simulink model "MPC_control_ID"  (R2018a)
settings: Solver=FixedStepAuto  StartTime=0  StopTime=Tend  FixedStep=0.001  RelTol=5e-3
model workspace (MAT data in the model file):
  A_mu = 10
  B_reff = 8.386
  Cz = 7766.25
  DCT_Param.Transmission.Ratios = [3.78 2.18 1.43 1.03 0.935 0.84]
  DCT_Param.Transmission.Shaft_Inertia_Odd = 0.0023
  DCT_Param.Transmission.Shaft_Inertia_Even = 0.0009
  DCT_Param.Transmission.Shaft_Inertia_Output = 0.008
  DCT_Param.Transmission.Gear_Inertia = 0.001
  DCT_Param.Transmission.Gear_Efficiency = 0.94
  DCT_Param.Transmission.Gear_Ang_Vel_Thr = 0.01
  DCT_Param.Transmission.Shaft_Velocity_Odd = 0
  DCT_Param.Transmission.Shaft_Velocity_Even = 0
  DCT_Param.Transmission.Shaft_Velocity_Output = 0
  DCT_Param.Transmission.Gear_Initial_Velocity = 0
  DCT_Param.Transmission.Abstract.Compliance = 100000
  DCT_Param.Transmission.Abstract.Damping = 10000
  DCT_Param.Transmission.Abstract.Ratio_Time_Const = 0.05
  DCT_Param.Transmission.Abstract.Shift_Gear_Delay = 25
  DCT_Param.Clutch.Torque_Radius = 130
  DCT_Param.Clutch.Num_Friction_Surfaces = 4
  DCT_Param.Clutch.Engagement_Piston_Area = 0.001
  DCT_Param.Clutch.Kinetic_Friction_Coeff = 0.3
  DCT_Param.Clutch.Static_Friction_Coeff = 0.31
  DCT_Param.Clutch.Derating_Factor = 1
  DCT_Param.Clutch.Clutch_Velocity_Tolerance = 0.001
  DCT_Param.Clutch.Threshold_Pressure = 1
  DCT_Param.Clutch.Drag_Torque_Coeff = 0
  DCT_Param.Dog_Clutch.Max_Torque = 1000
  DCT_Param.Dog_Clutch.Teeth_Mean_Radius = 50
  DCT_Param.Dog_Clutch.Tooth_Height = 10
  DCT_Param.Dog_Clutch.Ring_Hub_Clearance = 3
  DCT_Param.Dog_Clutch.Ring_Stop_Stiffness = 1000000
  DCT_Param.Dog_Clutch.Ring_Stop_Damping = 1000
  DCT_Param.Dog_Clutch.Shift_Linkage_Damping = 100
  DCT_Param.Dog_Clutch.Max_Engage_Velocity = 1000000
  DCT_Param.Dog_Clutch.Tooth_Engage_Overlap = 3
  DCT_Param.Vehicle.Mass = 1600
  DCT_Param.Vehicle.Wheels_Per_Axle = 2
  DCT_Param.Vehicle.Distance_CG_FrontAxle = 1.7
  DCT_Param.Vehicle.Distance_CG_RearAxle = 2
  DCT_Param.Vehicle.Distance_CG_Ground = 0.5
  DCT_Param.Vehicle.Frontal_Area = 3
  DCT_Param.Vehicle.Aero_Drag_Coeff = 0.4
  DCT_Param.Vehicle.Initial_Velocity = 0
  DCT_Param.Vehicle.Final_Drive_Ratio = 3.7
  DCT_Param.Vehicle.Final_Drive_Efficiency = 0.86
  DCT_Param.Vehicle.Final_Drive_Vel_Thresh = 0.01
  DCT_Param.Vehicle.Side_Shaft_Inertia = 0.01
  DCT_Param.Vehicle.Side_Shaft_Initial_Velocity = 0
  DCT_Param.Vehicle.Tire.Radius = 0.312
  DCT_Param.Vehicle.Tire.Inertia = 0.5
  DCT_Param.Vehicle.Tire.Initial_Velocity = 0
  DCT_Param.Vehicle.Tire.Slip_Vel_Thresh = 0.1
  DCT_Param.Vehicle.Tire.Nominal_Vertical_Load = 4000
  DCT_Param.Vehicle.Tire.C_Coeff = 1.685
  DCT_Param.Vehicle.Tire.D_Coeff = [1.21 -0.037]
  DCT_Param.Vehicle.Tire.E_Coeff = [0.344 0.095 -0.02 0]
  DCT_Param.Vehicle.Tire.BCD_Coeff = [21.51 -0.163 0.245]
  DCT_Param.Vehicle.Tire.H_Coeff = [-0.002 0.002]
  DCT_Param.Vehicle.Tire.V_Coeff = [0 0]
  DCT_Param.ICE.Max_Power = 100000
  DCT_Param.ICE.Speed_At_Max_Power = 5500
  DCT_Param.ICE.Max_Speed = 7000
  DCT_Param.ICE.Stall_Speed = 200
  DCT_Param.ICE.Shaft_Inertia = 0.2
  DCT_Param.ICE.Initial_Velocity = 800
  DCT_Param.ICE.Idle_Ref_Spd = 800
  DCT_Param.ICE.Engine_Time_Constant = 0.2
  DCT_Param.ICE.Initial_Normalized_Throttle = 0
  DCT_Param.ICE.Speed_Threshold = 20
  DCT_Param.ICE.FC.Speed_Vector = [0 368.421052632 736.842105263 1105.26315789 1473.68421053 1842.10526316 2210.52631579 2578.94736842 2947.36842105 3315.78947368 3684.21052632 4052.63157895 4421.05263158 4789.47368421 5157.89473684 5526.31578947 5894.73684211 6263.15789474 6631.57894737 7000]
  DCT_Param.ICE.FC.Torque_Vector = [0 10.5263157895 21.0526315789 31.5789473684 42.1052631579 52.6315789474 63.1578947368 73.6842105263 84.2105263158 94.7368421053 105.263157895 115.789473684 126.315789474 136.842105263 147.368421053 157.894736842 168.421052632 178.947368421 189.473684211 200]
  DCT_Param.ICE.FC.Consumption_Table = [0.262945178015 0.225304787522 0.201465019624 0.191425874321 0.195187351614 0.212749451502 0.244112173984 0.289275519063 0.348239486736 0.421004077004 0.507569289868 0.607935125326 ... (400 elements, 20x20)]
  DCT_Param.Shift_Map_Example.Pedal_Positions = [0.1 0.4 0.5 0.9]
  DCT_Param.Shift_Map_Example.Upshift_Speeds = [11  20  26  34.5  43; 14  26  35  44.5  55; 17  31  42  52.5  65; 21  39  52  66.5  80]
  DCT_Param.Shift_Map_Example.Downshift_Speeds = [8.9  17  23.6  32.4  40.8; 11.5  22.7  32  41.6  52.2; 14  27  38.1  50  62; 18  33  48  62.6  76.2]
  DCT_Param.Shift_Map_ORIG.Pedal_Positions = [0.1 0.4 0.5 0.9]
  DCT_Param.Shift_Map_ORIG.Upshift_Speeds = [11.5  23.5  35.5  45.5  55.5; 14.5  26.5  38.5  48.5  58.5; 17.5  29.5  41.5  51.5  61.5; 20.5  32.5  44.5  54.5  64.5]
  DCT_Param.Shift_Map_ORIG.Downshift_Speeds = [8.5  20.5  32.5  42.5  52.5; 11.5  23.5  35.5  45.5  55.5; 14.5  26.5  38.5  48.5  58.5; 17.5  29.5  41.5  51.5  61.5]
  DCT_Param.Shift_Map_OPT.Pedal_Positions = [0.1 0.4 0.5 0.9]
  DCT_Param.Shift_Map_OPT.Upshift_Speeds = [17.8469  29.8469  35.8159  41.2981  46.3004; 19.2469  33.9778  43.9778  53.9778  63.9778; 24.5469  41.9778  62.1778  78.5778  106.9778; 27.5469  59.3778  99.0445  109.0445  119.0445]
  DCT_Param.Shift_Map_OPT.Downshift_Speeds = [14.8469  26.8469  32.8159  38.2981  43.3004; 16.2469  30.9778  40.9778  50.9778  60.9778; 21.5469  38.9778  59.1778  75.5778  103.9778; 24.5469  56.3778  96.0445  106.0445  116.0445]
  DCT_Param.Shift_Map.Pedal_Positions = [0.1 0.4 0.5 0.9]
  DCT_Param.Shift_Map.Upshift_Speeds = [11.5  23.5  35.5  45.5  55.5; 14.5  26.5  38.5  48.5  58.5; 17.5  29.5  41.5  51.5  61.5; 20.5  32.5  44.5  54.5  64.5]
  DCT_Param.Shift_Map.Downshift_Speeds = [8.5  20.5  32.5  42.5  52.5; 11.5  23.5  35.5  45.5  55.5; 14.5  26.5  38.5  48.5  58.5; 17.5  29.5  41.5  51.5  61.5]
  DCT_Param.Control.Clutch.Min_Lock_Pressure = 2000000
  DCT_Param.Control.Clutch.Max_Lock_Pressure = 5000000
  DCT_Param.Control.Clutch.Max_Unlock_Pressure = 500000
  DCT_Param.Control.Engine_Start_RPM = 800
  DCT_Param.Control.Engine_Stop_RPM = 790
  DCT_Param.Control.Mode_Logic_TS = 0.1
  DCT_Param.Control.ICE.Kp = 0.02
  DCT_Param.Control.ICE.Ki = 0.01
  DCT_Param.Control.Gen.Kp = 10
  DCT_Param.Control.Gen.Ki = 3
  DCT_Param.Control.Mot.Kp = 500
  DCT_Param.Control.Mot.Ki = 300
  DCT_Param.Control.Veh_Spd.Kp = 0.02
  DCT_Param.Control.Veh_Spd.Ki = 0.04
  DCT_Param.Driver.Kp = 400
  DCT_Param.Driver.Ki = 0.001
  DCT_Param.Driver.Pedal_Filter_Const = 0.01
  DCT_Param.Dog_Clutches.Pulse_Delay = 50
  DCT_Param.Dog_Clutches.Pulse_Length = 20
  DCT_Param.Animation.Teeth_Ratios = [0.338461538462 0.555555555556 0.916666666667 0.96 1.17948717949 1.92307692308]
  DCT_Param.Animation.Teeth_Ratios_Reverse = [0.458333333333 0.75]
  DCT_Param.Shift_Map_OPT506.Pedal_Positions = [0.1 0.4 0.5 0.9]
  DCT_Param.Shift_Map_OPT506.Upshift_Speeds = [18  30.2  48.3  67.3322  77.3429; 20.1  36.85  66.6178  76.7537  86.7537; 21.1  40.25  71.0189  81.0189  91.7873; 24.1  63.75  80.7523  105.9489  115.9489]
  DCT_Param.Shift_Map_OPT506.Downshift_Speeds = [15  27.2  45.3  64.3322  74.3429; 17.1  33.85  63.6178  73.7537  83.7537; 18.1  37.25  68.0189  78.0189  88.7873; 21.1  60.75  77.7523  102.9489  112.9489]
  DCT_Param.Shift_Map_OPTAbsRea176.Pedal_Positions = [0.1 0.4 0.5 0.9]
  DCT_Param.Shift_Map_OPTAbsRea176.Upshift_Speeds = [17.8469  29.8469  35.7875  44.0901  49.4243; 18.9219  34.1312  45.8256  59.7585  69.7585; 32.1719  43.4585  53.51  103.2151  114.6401; 35.1719  59.2585  99.5217  109.5217  119.5217]
  DCT_Param.Shift_Map_OPTAbsRea176.Downshift_Speeds = [14.8469  26.8469  32.7875  41.0901  46.4243; 15.9219  31.1312  42.8256  56.7585  66.7585; 29.1719  40.4585  50.51  100.2151  111.6401; 32.1719  56.2585  96.5217  106.5217  116.5217]
  D_reff = 0.25826
  Downshift_Speeds = [9.5625  23.0625  36.5625  47.8125  59.0625  68.90625  78.75; 12.9375  26.4375  39.9375  51.1875  62.4375  72.84375  83.25; 16.3125  29.8125  43.3125  54.5625  65.8125  76.78125  87.75; 19.6875  33.1875  46.6875  57.9375  69.1875  80.71875  92.25]
  Pedal_Positions = [0.1 0.4 0.5 0.9]
  SUS.Stiffness = 24000
  SUS.Damping.Constant = 1262
  SUS.Damping.Rebound = [4040 4950 2883 2043]
  SUS.Damping.Compression = [3600 3420 1863 1472]
  SUS.PistonSpeed = [0.05 0.1 0.3 0.6]
  SUS.UnsprungMass.Fr = 21.0693333333
  SUS.UnsprungMass.Rr = 21.0693333333
  Upshift_Speeds = [12.9375  26.4375  39.9375  51.1875  62.4375  72.84375  83.25; 16.3125  29.8125  43.3125  54.5625  65.8125  76.78125  87.75; 19.6875  33.1875  46.6875  57.9375  69.1875  80.71875  92.25; 33  52.5  77.25  100.5  138.75  161.875  185]
  VEH.Mass = 1181
  VEH.StaticNormalFrontLoad.FR = 264.666666667
  VEH.StaticNormalFrontLoad.FL = 264.666666667
  VEH.StaticNormalRearLoad.RR = 322
  VEH.StaticNormalRearLoad.RL = 322
  VEH.WheelBase = 3.075
  VEH.FrontAxlePositionfromCG = 1.515
  VEH.RearAxlePositionfromCG = 1.504
  VEH.HeightCG = 0.134
  VEH.FrontalArea = 2.11
  VEH.DragCoefficient = 0.33
  VEH.NumberOfWheelsPerAxle = 2
  VEH.Thread.FR = 1.705
  VEH.Thread.RR = 1.705
  VEH.PitchMomentInertia = 1922.66666667
  VEH.RollMomentInertia = 432.333333333
  VEH.YawMomentInertia = 2066
  VEH.SteeringRatio = 18
  VEH.TrackWidth = 1.922
  VEH.SprungMass = 1096.72266667
  VEH.InitialLongPosition = 0
  VEH.InitialLatPosition = 3.125
  VEH.InitialVertPosition = 0.0111
  VEH.InitialRollAngle = 0
  VEH.InitialPitchAngle = -0.000732
  VEH.InitialYawAngle = 0
  VEH.InitialLongVel = 0
  VEH.InitialLatVel = 0
  VEH.InitialVertVel = 0
  VEH.InitialRollRate = 0
  VEH.InitialPitchRate = 0
  VEH.InitialYawRate = 0
  V_o = 16.7
  V_xlow = 1
  WH.Tire.Radius.Front = 0.384
  WH.Tire.Radius.Rear = 0.401
  WH.Tire.Sidewall = 0.245
  WH.Tire.RollingResistCoeff = 0.0103
  WH.Tire.Magic.B = 10
  WH.Tire.Magic.C = 1.9
  WH.Tire.Magic.D = 1
  WH.Tire.Magic.E = 0.97
  WH.Tire.Magic.Bx = 12
  WH.Tire.Magic.Cx = 1.9
  WH.Tire.Magic.Dx = 0.72
  WH.Tire.Magic.Ex = 0.95
  WH.Tire.Magic.By = 12
  WH.Tire.Magic.Cy = 1.3
  WH.Tire.Magic.Dy = 0.75
  WH.Tire.Magic.Ey = 0.2
  WH.Tire.Front.Ky = 40000
  WH.Tire.Rear.Ky = 40000
  WH.Tire.Kz = 320000
  WH.Tire.Damping = 100
  WH.Inertia = 1.00333333333
  WH.Mass = 11.4333333333
  WH.DampingCoefficient = 0.01
  WH.VelocityTol = 0.1
  a = 1.4
  alpha_max = 1.5
  alpha_min = -1.5
  b = 1.8
  c_zo = 209651
  epsilon = 0.1
  h = 0.134
  path.ISO3888p2.x = [0 2 12 25.5 36.5 49 61]
  path.ISO3888p2.y = [0 0 0 3.725 3.725 0 0]
  path.ISO3888p2.ylb = [1.225 1.225 1.225 4.725 4.725 1.5 1.5]
  path.ISO3888p2.yrb = [-1.225 -1.225 -1.225 2.225 2.225 -1.5 -1.5]
  path.CUSC.x = [10.668 21.336 36.576 54.864 73.152]
  path.CUSC.y = [0 0 5.1816 0 0]
  path.CUSC.ylb = [1.2192 1.2192 7.0104 1.8288 1.8288]
  path.CUSC.yrb = [-1.2192 -1.2192 3.3528 -1.8288 -1.8288]
  pio = 220000
  q_Fcx = 0
  q_Fz2 = 15.4
  q_Fzy = 0
  q_reo = 0.9974
  q_sx1 = -0.007764
  q_sx10 = 0.2824
  q_sx11 = 5.349
  q_sx12 = 0
  q_sx13 = 0
  q_sx14 = 0
  q_sx2 = 1.1915
  q_sx3 = 0.013948
  q_sx4 = 4.912
  q_sx5 = 1.02
  q_sx6 = 22.83
  q_sx7 = 0.7104
  q_sx8 = -0.023393
  q_sx9 = 0.6581
  q_sy1 = 0.00702
  q_sy2 = 0
  q_sy3 = 0.001515
  q_sy4 = 8.514e-05
  q_sy5 = 0
  q_sy6 = 0
  q_sy7 = 0.9008
  q_sy8 = -0.4089
  q_v1 = 0.0007742
  q_v2 = 0.04667
  r_Bx1 = 12.531
  r_Bx2 = 9.532
  r_Bx3 = 0
  r_By1 = 10.615
  r_By2 = 7.705
  r_By3 = 3.433e-06
  r_By4 = 0
  r_Cx1 = 1.019
  r_Cy1 = 1.0585
  r_Ex1 = -0.4487
  r_Ex2 = -0.4726
  r_Ey1 = 0.3132
  r_Ey2 = 7.63e-06
  r_Hx1 = 0.0002374
  r_Hy1 = 0.011646
  r_Hy2 = 7.63e-06
  r_Vy1 = 0.05654
  r_Vy2 = 7.63e-06
  r_Vy3 = 0
  r_Vy4 = 99.9
  r_Vy5 = 2
  r_Vy6 = 15.814
  r_o = 0.3135
  vehWidth = 2
  w = 1
undefined symbols (not defined in the file): F, Gd, Hd, JE, JF_part, Ld, M, Np, ro, Tf, Ts, U_max, U_min, XYplot
libraries: simulink x5, sim3dlib x2, autolibutils x1, vehdynlibviscommon x1
(part 1 of 2)
settings Model: ModifiedByFormat=The MathWorks, Inc.  Creator=The MathWorks, Inc.  LastModifiedBy=The MathWorks, Inc.
settings SolverCC: ZeroCrossAlgorithm=Adaptive  DecoupledContinuousIntegration=on  MinimalZcImpactIntegration=on
settings DebuggingCC: SignalInfNanChecking=error  ArtificialAlgebraicLoopMsg=none  IgnoredZcDiagnostic=none  ModelReferenceExtraNoncontSigs=none
settings ModelReferenceCC: UpdateModelReferenceTargets=IfOutOfDate  EnableParallelModelReferenceBuilds=on  ModelReferenceMinAlgLoopOccurrences=on  PropagateSignalLabelsOutOfModel=off
settings RTWCC: BuildConfiguration=Faster Runs

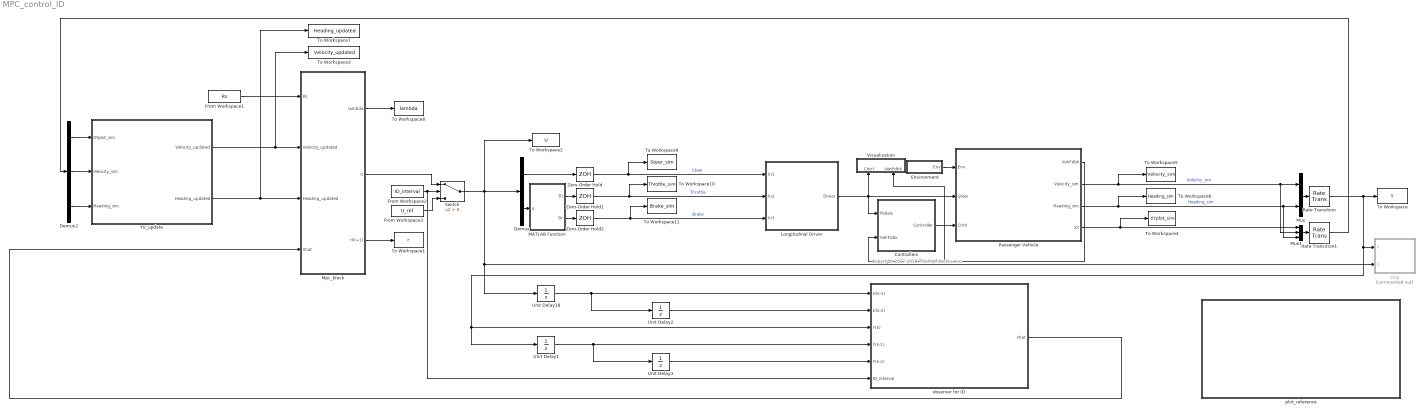
== system MPC_control_ID ==
  note: Copyright 2017-2018 The MathWorks, Inc.
  Controllers : Subsystem
      mask Display: image('SystemControllers.png')
  Demux : Demux  Outputs=2
  Demux2 : Demux  Outputs=3
  Environment : Subsystem  TreatAsAtomicUnit=on
      mask Display: disp('Environment')
  From Workspace1 : FromWorkspace  VariableName=Rs  SampleTime=Ts
  From Workspace2 : FromWorkspace  VariableName=ID_interval  SampleTime=Ts
  From Workspace3 : FromWorkspace  VariableName=U_ref  SampleTime=Ts
  Longitudinal Driver : Subsystem  SystemSampleTime=Tf  VariantControl=0
      mask Display: image('longitudinal_driver_pedals.png');
  MATLAB Function : MATLAB Function  TreatAsAtomicUnit=on  SystemSampleTime=Ts
  Mpc_block : Subsystem  TreatAsAtomicUnit=on  SystemSampleTime=Ts
  Mux : Mux  Inputs=2
  Mux1 : Mux  Inputs=3
  Passenger Vehicle : Subsystem  TreatAsAtomicUnit=on
      settings: MinAlgLoopOccurrences=on
      mask Display: image('PassengerVehicle.png')
  Rate Transition : RateTransition  OutPortSampleTime=Ts
  Rate Transition1 : RateTransition  OutPortSampleTime=Ts
  Switch : Switch  Criteria=u2 > Threshold
  To Workspace : ToWorkspace  VariableName=Y  SampleTime=Ts
  To Workspace1 : ToWorkspace  VariableName=r  SampleTime=Ts
  To Workspace10 : ToWorkspace  VariableName=Throttle_sim  SampleTime=Ts
  To Workspace11 : ToWorkspace  VariableName=Brake_sim  SampleTime=Ts
  To Workspace2 : ToWorkspace  VariableName=U  SampleTime=Ts
  To Workspace3 : ToWorkspace  VariableName=Velocity_updated  SampleTime=Ts
      settings: Save2DSignal=2-D array (concatenate along first dimension)
  To Workspace4 : ToWorkspace  VariableName=XYplot_sim  SampleTime=Ts
  To Workspace5 : ToWorkspace  VariableName=Velocity_sim  SampleTime=Ts
  To Workspace6 : ToWorkspace  VariableName=Heading_sim  SampleTime=Ts
  To Workspace7 : ToWorkspace  VariableName=Heading_updated  SampleTime=Ts
      settings: Save2DSignal=2-D array (concatenate along first dimension)
  To Workspace8 : ToWorkspace  VariableName=lambda  SampleTime=Ts
  To Workspace9 : ToWorkspace  VariableName=Steer_sim  SampleTime=Ts
  Unit Delay1 : UnitDelay  InitialCondition=ro  SampleTime=Ts
  Unit Delay18 : UnitDelay  InitialCondition=[0;0]  SampleTime=Ts
  Unit Delay2 : UnitDelay  InitialCondition=[0;0]  SampleTime=Ts
  Unit Delay3 : UnitDelay  InitialCondition=ro  SampleTime=Ts
  Visualization : Subsystem  TreatAsAtomicUnit=on
      mask Display: disp('Visualization')
  YV_update : Subsystem  TreatAsAtomicUnit=on
  Zero-Order Hold : ZeroOrderHold  SampleTime=Tf
  Zero-Order Hold1 : ZeroOrderHold  SampleTime=Tf
  Zero-Order Hold2 : ZeroOrderHold  SampleTime=Tf
  observer for ID : Subsystem
  plot_reference : Subsystem
      settings: MinAlgLoopOccurrences=on
  stop : Subsystem  Commented=on
  wires:
  Longitudinal Driver/1(Driver) -> Passenger Vehicle/2(Steer), Controllers/1(Pedals), Visualization/1(Cntrl)
  Environment/1(Env) -> Passenger Vehicle/1(Env)
  Controllers/1(Controller) -> Passenger Vehicle/3(Cntrl)
  Passenger Vehicle/1(VehFdbk) -> Controllers/2(VehFdbk), Visualization/2(VehFdbk)
  Demux/1 -> Zero-Order Hold/1
  MATLAB Function/1(Th) -> Zero-Order Hold1/1
  MATLAB Function/2(Br) -> Zero-Order Hold2/1
  Passenger Vehicle/3(Heading_sim) -> To Workspace6/1, Mux/2, Mux1/3  "Heading_sim"
  Mux/1 -> Rate Transition/1
  Demux/2 -> MATLAB Function/1(u)
  Zero-Order Hold/1 -> To Workspace9/1, Longitudinal Driver/1(In1)  "Steer"
  Zero-Order Hold1/1 -> To Workspace10/1, Longitudinal Driver/2(In2)  "Throttle"
  Zero-Order Hold2/1 -> To Workspace11/1, Longitudinal Driver/3(In3)  "Brake"
  Passenger Vehicle/2(Velocity_sim) -> To Workspace5/1, Mux/1, Mux1/2  "Velocity_sim"
  YV_update/2(Heading_updated) -> Mpc_block/3(Heading_updated), To Workspace7/1
  YV_update/1(Velocity_updated) -> Mpc_block/2(Velocity_updated), To Workspace3/1
  Demux2/2 -> YV_update/2(Velocity_sim)
  Mux1/1 -> Rate Transition1/1
  Demux2/1 -> YV_update/1(XYplot_sim)
  Demux2/3 -> YV_update/3(Heading_sim)
  Rate Transition1/1 -> Demux2/1
  From Workspace1/1 -> Mpc_block/1(Rs)
  Passenger Vehicle/4(XY) -> To Workspace4/1, Mux1/1
  observer for ID/1(xhat) -> Mpc_block/4(Xhat)
  Rate Transition/1 -> stop/1(Y), Unit Delay1/1, observer for ID/3(Y(k)), To Workspace/1
  Mpc_block/1(lambda) -> To Workspace8/1
  From Workspace2/1 -> Switch/2, observer for ID/6(ID_interval)
  Mpc_block/2(U) -> Switch/1
  Switch/1 -> To Workspace2/1, Demux/1, stop/2(U), Unit Delay18/1
  Unit Delay18/1 -> Unit Delay2/1, observer for ID/1(U(k-1))
  Unit Delay1/1 -> Unit Delay3/1, observer for ID/4(Y(k-1))
  Mpc_block/3(r(k+1)) -> To Workspace1/1
  Unit Delay2/1 -> observer for ID/2(U(k-2))
  Unit Delay3/1 -> observer for ID/5(Y(k-2))
  From Workspace3/1 -> Switch/3

== system MPC_control_ID/Controllers ==
  Pedals : Inport
  VehFdbk : Inport  Port=2
  Brake Controller : Subsystem
  Bus Creator : BusCreator  Inputs=1
  Bus Creator1 : BusCreator  Inputs=1
  Bus Creator2 : BusCreator  Inputs=1
  Bus Creator3 : BusCreator  Inputs=3
  Bus Selector : BusSelector  OutputSignals=Body.xdot,Wheels.kappa
  Bus Selector1 : BusSelector  OutputSignals=Driveline.EngSpd,Driveline.PropShftSpd
  Bus Selector2 : BusSelector  OutputSignals=Accel,Brake
  ECU : Subsystem
  Transmission Controller : Subsystem
  Controller : Outport
  wires:
  Transmission Controller/1(Gear) -> Bus Creator1/1  "GearCmd"
  Bus Selector/2 -> Brake Controller/3(kappa)  "<kappa>"
  ECU/1(Trq Cmd) -> Bus Creator/1  "EngTrqCmd"
  Brake Controller/1(PCmd) -> Bus Creator2/1  "PrsCmd"
  VehFdbk/1 -> Bus Selector/1, Bus Selector1/1
  Bus Selector/1 -> Brake Controller/2(xdot)  "<xdot>"
  Bus Selector1/1 -> Transmission Controller/2(EngSpd)  "<EngSpd>"
  Bus Selector1/2 -> Transmission Controller/3(PropShaftSpd)  "<PropShftSpd>"
  Pedals/1 -> Bus Selector2/1
  Bus Selector2/1 -> Transmission Controller/1(Acc), ECU/1(<Accel>)  "<Accel>"
  Bus Selector2/2 -> Brake Controller/1(BrkPrsCmd)  "<Brake>"
  Bus Creator/1 -> Bus Creator3/1  "ECU"
  Bus Creator1/1 -> Bus Creator3/2  "Transmission"
  Bus Creator2/1 -> Bus Creator3/3  "Brake"
  Bus Creator3/1 -> Controller/1  "Controller"

== system MPC_control_ID/Environment ==
  Bus Creator : BusCreator  Inputs=4
  Bus Creator1 : BusCreator  Inputs=2
  Bus Creator2 : BusCreator  Inputs=4
  Bus Creator3 : BusCreator  Inputs=2
  Constant1 : Constant  Value=zeros(4,1)
  Constant3 : Constant  Value=0
  Constant4 : Constant  Value=0
  Constant5 : Constant  Value=0
  Demux : Demux
  Demux1 : Demux
  Friction : Constant  Value=ones(4,1).*1
  Vector Concatenate : Concatenate  NumInputs=3
  Env : Outport
  wires:
  Constant1/1 -> Demux/1
  Bus Creator2/1 -> Bus Creator3/2  "mu"
  Bus Creator/1 -> Bus Creator3/1  "z"
  Demux/2 -> Bus Creator/2  "G_FR_z"
  Demux/3 -> Bus Creator/3  "G_RL_z"
  Constant5/1 -> Vector Concatenate/3  "Z"
  Demux/1 -> Bus Creator/1  "G_FL_z"
  Vector Concatenate/1 -> Bus Creator1/1  "Wind"
  Constant3/1 -> Vector Concatenate/1  "X"
  Demux/4 -> Bus Creator/4  "G_RR_z"
  Constant4/1 -> Vector Concatenate/2  "Y"
  Demux1/3 -> Bus Creator2/3  "mu_RL"
  Demux1/4 -> Bus Creator2/4  "mu_RR"
  Demux1/2 -> Bus Creator2/2  "mu_FR"
  Demux1/1 -> Bus Creator2/1  "mu_FL"
  Friction/1 -> Demux1/1
  Bus Creator3/1 -> Bus Creator1/2  "Gnd"
  Bus Creator1/1 -> Env/1

== system MPC_control_ID/Longitudinal Driver ==
  In1 : Inport  SampleTime=Tf
  In2 : Inport  Port=2  SampleTime=Tf
  In3 : Inport  Port=3  SampleTime=Tf
  Bus Creator1 : BusCreator  Inputs=3
  Driver : Outport
  wires:
  Bus Creator1/1 -> Driver/1
  In2/1 -> Bus Creator1/2  "Accel"
  In3/1 -> Bus Creator1/3  "Brake"
  In1/1 -> Bus Creator1/1  "Steer"

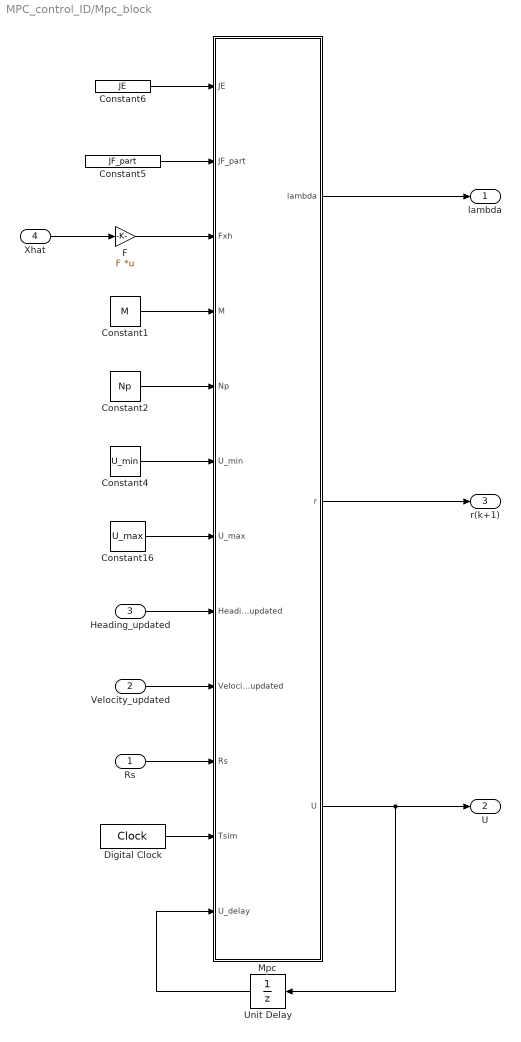
== system MPC_control_ID/Mpc_block ==
  Rs : Inport  SampleTime=Ts  LockScale=on
  Velocity_updated : Inport  Port=2  SampleTime=Ts
  Heading_updated : Inport  Port=3  SampleTime=Ts  LockScale=on
  Xhat : Inport  Port=4
  Constant1 : Constant  Value=M  VectorParams1D=off  SampleTime=-1
  Constant16 : Constant  Value=U_max  VectorParams1D=off  SampleTime=-1
  Constant2 : Constant  Value=Np  SampleTime=-1
  Constant4 : Constant  Value=U_min  VectorParams1D=off  SampleTime=-1
  Constant5 : Constant  Value=JF_part  VectorParams1D=off  SampleTime=-1
  Constant6 : Constant  Value=JE  VectorParams1D=off  SampleTime=-1
  Digital Clock : DigitalClock  SampleTime=Ts
  F : Gain  Gain=F  Multiplication=Matrix(K*u) (u vector)
  Mpc : MATLAB Function  TreatAsAtomicUnit=on  SystemSampleTime=Ts
  Unit Delay : UnitDelay  InitialCondition=[0;0]  SampleTime=Ts
  lambda : Outport
  U : Outport  Port=2
  r(k+1) : Outport  Port=3
  wires:
  Unit Delay/1 -> Mpc/12(U_delay)
  Heading_updated/1 -> Mpc/8(Heading_updated)
  Constant1/1 -> Mpc/4(M)
  Mpc/3(U) -> U/1, Unit Delay/1
  Constant2/1 -> Mpc/5(Np)
  Xhat/1 -> F/1
  Rs/1 -> Mpc/10(Rs)
  Constant4/1 -> Mpc/6(U_min)
  Velocity_updated/1 -> Mpc/9(Velocity_updated)
  Constant6/1 -> Mpc/1(JE)
  Mpc/2(r) -> r(k+1)/1
  Digital Clock/1 -> Mpc/11(Tsim)
  Constant16/1 -> Mpc/7(U_max)
  Mpc/1(lambda) -> lambda/1
  F/1 -> Mpc/3(Fxh)
  Constant5/1 -> Mpc/2(JF_part)

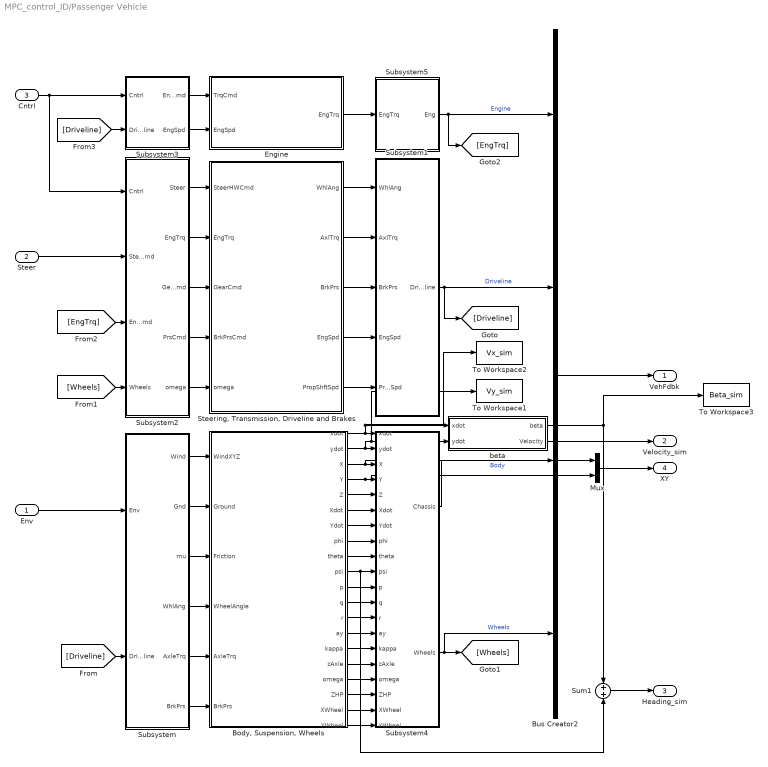
== system MPC_control_ID/Passenger Vehicle ==
  Env : Inport
  Steer : Inport  Port=2
  Cntrl : Inport  Port=3
  "Body, Suspension, Wheels" : Subsystem  Variant=on  OverrideUsingVariant=1
  Bus Creator2 : BusCreator  Inputs=4
  Engine : Subsystem  Variant=on  OverrideUsingVariant=0
  Mux : Mux  Inputs=2
  "Steering, Transmission, Driveline and Brakes" : Subsystem  Variant=on  OverrideUsingVariant=0
  Subsystem : Subsystem
  Subsystem1 : Subsystem
  Subsystem2 : Subsystem
  Subsystem3 : Subsystem
  Subsystem4 : Subsystem
  Subsystem5 : Subsystem
  Sum1 : Sum
  To Workspace1 : ToWorkspace  VariableName=Vy_sim  SampleTime=Ts
  To Workspace2 : ToWorkspace  VariableName=Vx_sim  SampleTime=Ts
  To Workspace3 : ToWorkspace  VariableName=Beta_sim  SampleTime=Ts
  beta : MATLAB Function  TreatAsAtomicUnit=on  SystemSampleTime=Tf
      settings: MinAlgLoopOccurrences=on
  VehFdbk : Outport
  Velocity_sim : Outport  Port=2
  Heading_sim : Outport  Port=3
  XY : Outport  Port=4
  wires:
  Bus Creator2/1 -> VehFdbk/1
  Env/1 -> Subsystem/1(Env)
  Subsystem1/1(Driveline) -> [Driveline], Bus Creator2/2  "Driveline"
  "Steering, Transmission, Driveline and Brakes"/1(WhlAng) -> Subsystem1/1(WhlAng)
  "Steering, Transmission, Driveline and Brakes"/2(AxlTrq) -> Subsystem1/2(AxlTrq)
  "Steering, Transmission, Driveline and Brakes"/3(BrkPrs) -> Subsystem1/3(BrkPrs)
  "Steering, Transmission, Driveline and Brakes"/4(EngSpd) -> Subsystem1/4(EngSpd)
  "Steering, Transmission, Driveline and Brakes"/5(PropShftSpd) -> Subsystem1/5(PropShftSpd)
  Steer/1 -> Subsystem2/2(SteerCmd)
  Cntrl/1 -> Subsystem3/1(Cntrl), Subsystem2/1(Cntrl)
  Subsystem2/1(Steer) -> "Steering, Transmission, Driveline and Brakes"/1(SteerHWCmd)
  Subsystem2/3(GearCmd) -> "Steering, Transmission, Driveline and Brakes"/3(GearCmd)
  Subsystem2/4(PrsCmd) -> "Steering, Transmission, Driveline and Brakes"/4(BrkPrsCmd)
  Subsystem2/5(omega) -> "Steering, Transmission, Driveline and Brakes"/5(omega)
  Engine/1(EngTrq) -> Subsystem5/1("EngTrq ")
  Subsystem2/2(EngTrq) -> "Steering, Transmission, Driveline and Brakes"/2(EngTrq)
  Subsystem3/1(EngTrqCmd) -> Engine/1(TrqCmd)
  Subsystem3/2(EngSpd) -> Engine/2(EngSpd)
  Subsystem4/1(Chassis) -> Bus Creator2/3  "Body"
  Subsystem4/2(Wheels) -> Bus Creator2/4, [Wheels]  "Wheels"
  Subsystem5/1(Eng) -> [EngTrq], Bus Creator2/1  "Engine"
  [Driveline] -> Subsystem/2(Driveline)
  [Wheels] -> Subsystem2/4(Wheels)
  [EngTrq] -> Subsystem2/3(EngTrqCmd)
  [Driveline] -> Subsystem3/2(Driveline)
  "Body, Suspension, Wheels"/19(XWheel) -> Subsystem4/19(XWheel)
  "Body, Suspension, Wheels"/11(p) -> Subsystem4/11(p)
  "Body, Suspension, Wheels"/12(q) -> Subsystem4/12(q)
  "Body, Suspension, Wheels"/7(Ydot) -> Subsystem4/7(Ydot)
  "Body, Suspension, Wheels"/13(r) -> Subsystem4/13(r)
  "Body, Suspension, Wheels"/16(zAxle) -> Subsystem4/16(zAxle)
  "Body, Suspension, Wheels"/8(phi) -> Subsystem4/8(phi)
  "Body, Suspension, Wheels"/3(X) -> Mux/1, Subsystem4/3(X)
  Subsystem/6(BrkPrs) -> "Body, Suspension, Wheels"/6(BrkPrs)
  "Body, Suspension, Wheels"/9(theta) -> Subsystem4/9(theta)
  "Body, Suspension, Wheels"/5(Z) -> Subsystem4/5(Z)
  Subsystem/3(mu) -> "Body, Suspension, Wheels"/3(Friction)
  "Body, Suspension, Wheels"/17(omega) -> Subsystem4/17(omega)
  Subsystem/4(WhlAng) -> "Body, Suspension, Wheels"/4(WheelAngle)
  "Body, Suspension, Wheels"/14(ay) -> Subsystem4/14(ay)
  Subsystem/1(Wind) -> "Body, Suspension, Wheels"/1(WindXYZ)
  Subsystem/2(Gnd) -> "Body, Suspension, Wheels"/2(Ground)
  "Body, Suspension, Wheels"/10(psi) -> Subsystem4/10(psi), Sum1/2
  "Body, Suspension, Wheels"/4(Y) -> Mux/2, Subsystem4/4(Y)
  Subsystem/5(AxleTrq) -> "Body, Suspension, Wheels"/5(AxleTrq)
  "Body, Suspension, Wheels"/18(ZHP) -> Subsystem4/18(ZHP)
  "Body, Suspension, Wheels"/20(YWheel) -> Subsystem4/20(YWheel)
  "Body, Suspension, Wheels"/6(Xdot) -> Subsystem4/6(Xdot)
  "Body, Suspension, Wheels"/15(kappa) -> Subsystem4/15(kappa)
  Mux/1 -> XY/1
  Sum1/1 -> Heading_sim/1
  beta/1(beta) -> To Workspace3/1, Sum1/1
  "Body, Suspension, Wheels"/2(ydot) -> To Workspace1/1, beta/2(ydot), Subsystem4/2(ydot)
  "Body, Suspension, Wheels"/1(xdot) -> To Workspace2/1, beta/1(xdot), Subsystem4/1(xdot)
  beta/2(Velocity) -> Velocity_sim/1

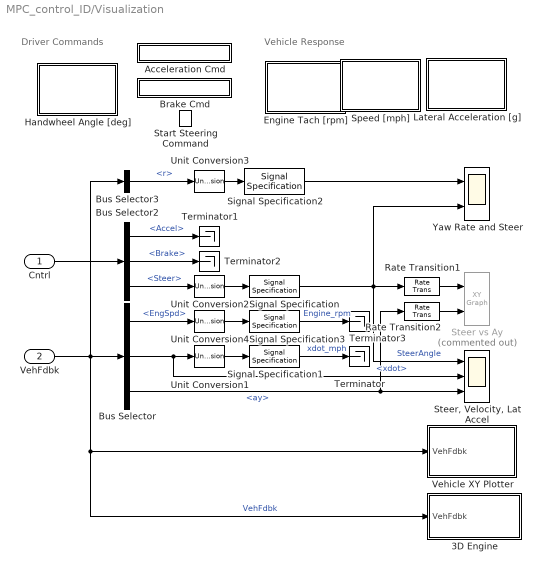
== system MPC_control_ID/Visualization ==
  note: Driver Commands
  note: Vehicle Response
  Cntrl : Inport
  VehFdbk : Inport  Port=2
  3D Engine : Subsystem  Variant=on  OverrideUsingVariant=0  mask(3D Engine){engine3D=Disabled, SceneDesc=Straight road, dt3D=.03}
      mask prompts: engine3D "3D Engine"; SceneDesc "Scene Description:"; dt3D "Engine frame rate, dt3D [s]:"
      mask help: This subsystem contains the interface blocks which permit the display of the vehicle in 3D virtual environment. Enable it to view the simulation progress, disable it to inhibit the display.
      mask init:
      | switch get_param(gcb,'engine3D')
      |     case 'Disabled'
      |         set_param(gcb,'OverrideUsingVariant','0')
      |     case 'Enabled'
      |        set_param(gcb,'OverrideUsingVariant','1')
      |     otherwise
      |        set_param(gcb,'OverrideUsingVariant','0')
      | end
      settings: AttributesFormatString=%<engine3D>
      mask Help: eval('vdynblkshelp(''vdynblksscenecameraray'')');
      mask TypeOptions engine3D: Enabled | Disabled
      mask Callback engine3D:
      | switch get_param(gcb,'engine3D')
      |     case 'Disabled'
      |         set_param(gcb,'OverrideUsingVariant','0')
      |     case 'Enabled'
      |        set_param(gcb,'OverrideUsingVariant','1')
      |     otherwise
      |        set_param(gcb,'OverrideUsingVariant','0')
      | end
      mask TypeOptions SceneDesc:
      | 3D Engine/Simulation 3D Engine
      | 1/SceneDesc
      mask Display: disp('3D Engine')
  Acceleration Cmd : Subsystem  DialogController=hmiCreateDDGDialog  IsWebBlock=on  mask(MWDashboardBlock){webBlockId=2ec56b20-76c2-4aac-ab3d-2dd24ca42fe8, webBlockType=lineargauge, ShowInLibBrowser=on, ShowInitialText=on, HMISrcModelName=[]}
      mask prompts: webBlockId "WebBlock Id"; webBlockType "WebBlock Type"; HMISrcModelName "Source Model"
      mask help: SimulinkHMI:dialogs:LinearGaugeDialogDesc
      mask Help: helpview([docroot '/mapfiles/simulink.map'], 'hmi_linear_gauge')
      mask Display:
      | if strcmp(get_param(bdroot(gcb),'BlockDiagramType'), 'library')
      |     image([(matlabroot) '/toolbox/simulink/hmi/icons/LinearGauge.png']);
      | end
  Brake Cmd : Subsystem  DialogController=hmiCreateDDGDialog  IsWebBlock=on  mask(MWDashboardBlock){webBlockId=d9917a9d-f04e-4f5f-9d8a-619b2f9adbbc, webBlockType=lineargauge, ShowInLibBrowser=on, ShowInitialText=on, HMISrcModelName=[]}
      mask prompts: webBlockId "WebBlock Id"; webBlockType "WebBlock Type"; HMISrcModelName "Source Model"
      mask help: SimulinkHMI:dialogs:LinearGaugeDialogDesc
      mask Help: helpview([docroot '/mapfiles/simulink.map'], 'hmi_linear_gauge')
      mask Display:
      | if strcmp(get_param(bdroot(gcb),'BlockDiagramType'), 'library')
      |     image([(matlabroot) '/toolbox/simulink/hmi/icons/LinearGauge.png']);
      | end
  Bus Selector : BusSelector  OutputSignals=Driveline.EngSpd,Body.xdot,Body.ay
  Bus Selector2 : BusSelector  OutputSignals=Accel,Brake,Steer
  Bus Selector3 : BusSelector  OutputSignals=Body.r
  Engine Tach [rpm] : Subsystem  DialogController=hmiCreateDDGDialog  IsWebBlock=on  mask(MWDashboardBlock){webBlockId=b43bb858-1bc3-4216-8222-68d06605e534, webBlockType=circulargauge, ShowInLibBrowser=on, ShowInitialText=on, HMISrcModelName=[]}
      mask prompts: webBlockId "WebBlock Id"; webBlockType "WebBlock Type"; HMISrcModelName "Source Model"
      mask help: SimulinkHMI:dialogs:CircularGaugeDialogDesc
      mask Help: helpview([docroot '/mapfiles/simulink.map'], 'hmi_gauge')
      mask Display:
      | if strcmp(get_param(bdroot(gcb),'BlockDiagramType'), 'library')
      |     image([(matlabroot) '/toolbox/simulink/hmi/icons/CircularGauge.png']);
      | end
  Handwheel Angle [deg] : Subsystem  DialogController=hmiCreateDDGDialog  IsWebBlock=on  mask(MWDashboardBlock){webBlockId=4efaf655-7637-4550-9856-9a687d94287b, webBlockType=semicirculargauge, ShowInLibBrowser=on, ShowInitialText=on, HMISrcModelName=[]}
      mask prompts: webBlockId "WebBlock Id"; webBlockType "WebBlock Type"; HMISrcModelName "Source Model"
      mask help: SimulinkHMI:dialogs:SemicircularGaugeDialogDesc
      mask Help: helpview([docroot '/mapfiles/simulink.map'], 'hmi_half_gauge')
      mask Display:
      | if strcmp(get_param(bdroot(gcb),'BlockDiagramType'), 'library')
      |     image([(matlabroot) '/toolbox/simulink/hmi/icons/SemicircularGauge.png']);
      | end
  Lateral Acceleration [g] : Subsystem  DialogController=hmiCreateDDGDialog  IsWebBlock=on  mask(MWDashboardBlock){webBlockId=4c84f06f-3c50-4c9f-a814-1d904b0076de, webBlockType=semicirculargauge, ShowInLibBrowser=on, ShowInitialText=on, HMISrcModelName=[]}
      mask prompts: webBlockId "WebBlock Id"; webBlockType "WebBlock Type"; HMISrcModelName "Source Model"
      mask help: SimulinkHMI:dialogs:SemicircularGaugeDialogDesc
      mask Help: helpview([docroot '/mapfiles/simulink.map'], 'hmi_half_gauge')
      mask Display:
      | if strcmp(get_param(bdroot(gcb),'BlockDiagramType'), 'library')
      |     image([(matlabroot) '/toolbox/simulink/hmi/icons/SemicircularGauge.png']);
      | end
  Rate Transition1 : RateTransition
  Rate Transition2 : RateTransition
  Signal Specification : SignalSpecification  Unit=deg
  Signal Specification1 : SignalSpecification  Unit=mph
  Signal Specification2 : SignalSpecification  Unit=deg/s
  Signal Specification3 : SignalSpecification  Unit=rpm
  Speed [mph] : Subsystem  DialogController=hmiCreateDDGDialog  IsWebBlock=on  mask(MWDashboardBlock){webBlockId=6d425e54-616c-4430-b762-4652b407af79, webBlockType=circulargauge, ShowInLibBrowser=on, ShowInitialText=on, HMISrcModelName=[]}
      mask prompts: webBlockId "WebBlock Id"; webBlockType "WebBlock Type"; HMISrcModelName "Source Model"
      mask help: SimulinkHMI:dialogs:CircularGaugeDialogDesc
      mask Help: helpview([docroot '/mapfiles/simulink.map'], 'hmi_gauge')
      mask Display:
      | if strcmp(get_param(bdroot(gcb),'BlockDiagramType'), 'library')
      |     image([(matlabroot) '/toolbox/simulink/hmi/icons/CircularGauge.png']);
      | end
  Start Steering Command : LampBlock  WebBlockId=3552  LabelPosition=Hide
  Steer vs Ay : simulink/Sinks/XY Graph  Commented=on  xmin=-300  xmax=300  ymin=-1.5  ymax=1.5  st=.1
  "Steer, Velocity, Lat Accel" : Scope  NumInputPorts=3
  Terminator{,1..3} (4 alike) : Terminator
  Unit Conversion{1..4} (4 alike) : UnitConversion
  Vehicle XY Plotter : Subsystem  mask(Vehicle XY Plotter){a=VEH.FrontAxlePositionfromCG, b=VEH.RearAxlePositionfromCG, w=VEH.TrackWidth, bufferSize=1024, pltDT=0.1}
      mask prompts: a "Distance to front axle from CG, a [m]:"; b "Distance to rear axle from CG, b [m]:"; w "Track width, w [m]:"; bufferSize "Path buffer sampe size, bufferSize []:"; pltDT "Plot update rate, pltDT [s]:"
      mask help: This block will display a MATLAB figure which indicates the vehicle path, current position and heading velocity.
      mask TypeOptions a: Vehicle XY Plotter/a
      mask TypeOptions b: Vehicle XY Plotter/b
      mask TypeOptions w: Vehicle XY Plotter/w
      mask TypeOptions bufferSize: Vehicle XY Plotter/bufferSize
  Yaw Rate and Steer : Scope  NumInputPorts=2
  wires:
  Unit Conversion3/1 -> Signal Specification2/1
  Bus Selector3/1 -> Unit Conversion3/1  "<r>"
  Signal Specification2/1 -> Yaw Rate and Steer/1
  Unit Conversion4/1 -> Signal Specification3/1
  Signal Specification3/1 -> Terminator3/1  "Engine_rpm"
  Signal Specification/1 -> Yaw Rate and Steer/2, Rate Transition1/1, "Steer, Velocity, Lat Accel"/1  "SteerAngle"
  Bus Selector2/3 -> Unit Conversion2/1  "<Steer>"
  Signal Specification1/1 -> Terminator/1  "xdot_mph"
  Unit Conversion1/1 -> Signal Specification1/1
  Bus Selector/3 -> Rate Transition2/1, "Steer, Velocity, Lat Accel"/3  "<ay>"
  Bus Selector2/1 -> Terminator1/1  "<Accel>"
  Rate Transition1/1 -> Steer vs Ay/1
  Unit Conversion2/1 -> Signal Specification/1
  Bus Selector/2 -> "Steer, Velocity, Lat Accel"/2, Unit Conversion1/1  "<xdot>"
  VehFdbk/1 -> Bus Selector3/1, Bus Selector/1, Vehicle XY Plotter/1(VehFdbk), 3D Engine/1(VehFdbk)  "VehFdbk"
  Cntrl/1 -> Bus Selector2/1
  Rate Transition2/1 -> Steer vs Ay/2
  Bus Selector/1 -> Unit Conversion4/1  "<EngSpd>"
  Bus Selector2/2 -> Terminator2/1  "<Brake>"

== system MPC_control_ID/YV_update ==
  XYplot_sim : Inport
  Velocity_sim : Inport  Port=2
  Heading_sim : Inport  Port=3
  Constant2 : Constant  Value=Ts  SampleTime=Ts
  From Workspace1 : FromWorkspace  VariableName=Tsim  SampleTime=Ts
  From Workspace3 : FromWorkspace  VariableName=XYplot_ref  SampleTime=Ts
  MATLAB Function2 : MATLAB Function  TreatAsAtomicUnit=on  SystemSampleTime=Ts
  Velocity_updated : Outport
  Heading_updated : Outport  Port=2
  wires:
  MATLAB Function2/1(Velocity_updated) -> Velocity_updated/1
  From Workspace3/1 -> MATLAB Function2/1(XYplot_ref)
  MATLAB Function2/2(Heading_updated) -> Heading_updated/1
  From Workspace1/1 -> MATLAB Function2/6(Tsim)
  XYplot_sim/1 -> MATLAB Function2/2(XYplot_sim)
  Velocity_sim/1 -> MATLAB Function2/3(Velocity_sim)
  Heading_sim/1 -> MATLAB Function2/4(Heading_sim)
  Constant2/1 -> MATLAB Function2/5(Ts)

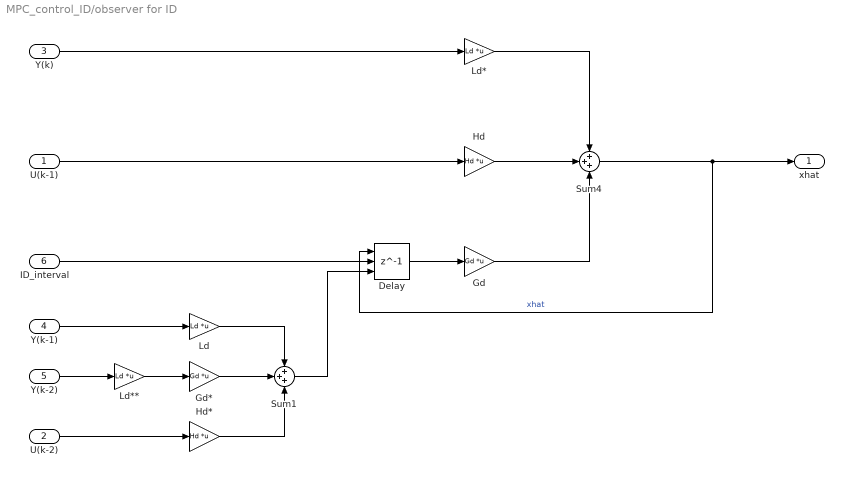
== system MPC_control_ID/observer for ID ==
  U(k-1) : Inport
  U(k-2) : Inport  Port=2
  Y(k) : Inport  Port=3
  Y(k-1) : Inport  Port=4
  Y(k-2) : Inport  Port=5
  ID_interval : Inport  Port=6
  Delay : Delay  DelayLength=1  InitialConditionSource=Input port  InitialCondition=0  ExternalReset=Rising  SampleTime=Ts
      settings: InputPortMap=u0,r5,p4
  Gd : Gain  Gain=Gd  Multiplication=Matrix(K*u) (u vector)
  Gd* : Gain  Gain=Gd  Multiplication=Matrix(K*u) (u vector)
  Hd : Gain  Gain=Hd  Multiplication=Matrix(K*u) (u vector)
  Hd* : Gain  Gain=Hd  Multiplication=Matrix(K*u) (u vector)
  Ld : Gain  Gain=Ld  Multiplication=Matrix(K*u) (u vector)
  Ld* : Gain  Gain=Ld  Multiplication=Matrix(K*u) (u vector)
  Ld** : Gain  Gain=Ld  Multiplication=Matrix(K*u) (u vector)
  Sum1 : Sum  Inputs=+++
  Sum4 : Sum  Inputs=+++
  xhat : Outport
  wires:
  Hd/1 -> Sum4/2
  Ld*/1 -> Sum4/1
  Gd/1 -> Sum4/3
  Sum4/1 -> Delay/1, xhat/1  "xhat"
  Delay/1 -> Gd/1
  Y(k-1)/1 -> Ld/1
  Y(k)/1 -> Ld*/1
  U(k-1)/1 -> Hd/1
  ID_interval/1 -> Delay/2
  Y(k-2)/1 -> Ld**/1
  Ld**/1 -> Gd*/1
  U(k-2)/1 -> Hd*/1
  Ld/1 -> Sum1/1
  Sum1/1 -> Delay/3
  Gd*/1 -> Sum1/2
  Hd*/1 -> Sum1/3

== system MPC_control_ID/plot_reference ==
  Clock : Clock
  Constant : Constant  Value=XYplot  SampleTime=Ts
  MATLAB Function1 : MATLAB Function  TreatAsAtomicUnit=on
  wires:
  Clock/1 -> MATLAB Function1/2(Tsim)
  Constant/1 -> MATLAB Function1/1(XYplot)

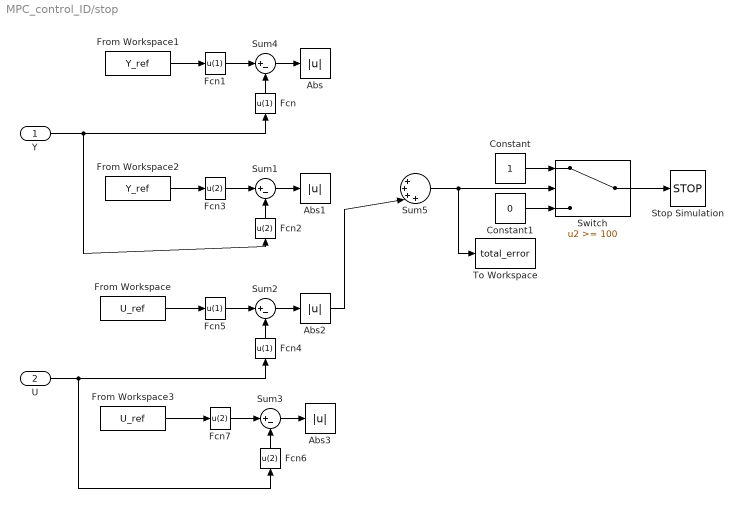
== system MPC_control_ID/stop ==
  Y : Inport
  U : Inport  Port=2
  Abs{,1..3} (4 alike) : Abs
  Constant : Constant
  Constant1 : Constant  Value=0
  Fcn{,1,4..5} (4 alike) : Fcn  Expr=u(1)
  Fcn{2..3,6..7} (4 alike) : Fcn  Expr=u(2)
  From Workspace : FromWorkspace  VariableName=U_ref  SampleTime=Ts
  From Workspace1 : FromWorkspace  VariableName=Y_ref  SampleTime=Ts
  From Workspace2 : FromWorkspace  VariableName=Y_ref  SampleTime=Ts
  From Workspace3 : FromWorkspace  VariableName=U_ref  SampleTime=Ts
  Stop Simulation : Stop
  Sum{1..4} (4 alike) : Sum  Inputs=|+-
  Sum5 : Sum  Inputs=|++++
  Switch : Switch  Threshold=100
  To Workspace : ToWorkspace  VariableName=total_error  SampleTime=Ts
  wires:
  From Workspace1/1 -> Fcn1/1
  Fcn/1 -> Sum4/2
  Fcn1/1 -> Sum4/1
  Sum4/1 -> Abs/1
  Fcn3/1 -> Sum1/1
  Sum1/1 -> Abs1/1
  Y/1 -> Fcn/1, Fcn2/1
  Fcn2/1 -> Sum1/2
  From Workspace2/1 -> Fcn3/1
  Fcn4/1 -> Sum2/2
  Sum2/1 -> Abs2/1
  Fcn5/1 -> Sum2/1
  From Workspace/1 -> Fcn5/1
  U/1 -> Fcn4/1, Fcn6/1
  Sum3/1 -> Abs3/1
  Fcn7/1 -> Sum3/1
  Fcn6/1 -> Sum3/2
  From Workspace3/1 -> Fcn7/1
  Constant/1 -> Switch/1
  Constant1/1 -> Switch/3
  Switch/1 -> Stop Simulation/1
  Sum5/1 -> Switch/2, To Workspace/1
  Abs2/1 -> Sum5/3

== system MPC_control_ID/Controllers/Brake Controller ==
  BrkPrsCmd : Inport
  xdot : Inport  Port=2
  kappa : Inport  Port=3
  Abs : Abs  ZeroCross=off
  Brake Pressure Control : Subsystem  Variant=on  OverrideUsingVariant=0
  Constant1 : Constant  Value=-20
  Gain3 : Gain
  Integrator2 : Integrator  LimitOutput=on  UpperSaturationLimit=1  LowerSaturationLimit=0
  Saturation : Saturate  UpperLimit=1  LowerLimit=0  ZeroCross=off
  Switch1 : Switch  Criteria=u2 > Threshold  Threshold=.1
  Vector Concatenate2 : Concatenate  NumInputs=4
  PCmd : Outport
  wires:
  Constant1/1 -> Switch1/3
  Gain3/1 -> Switch1/1
  Saturation/1 -> Brake Pressure Control/3(<Kappa>)  "Kappa"
  Brake Pressure Control/1(PCmd) -> PCmd/1
  kappa/1 -> Abs/1
  Integrator2/1 -> Vector Concatenate2/4, Vector Concatenate2/3, Vector Concatenate2/2, Vector Concatenate2/1
  xdot/1 -> Brake Pressure Control/2(xdot)
  Abs/1 -> Saturation/1
  Vector Concatenate2/1 -> Brake Pressure Control/1(Pref)  "Reference P"
  BrkPrsCmd/1 -> Switch1/2, Gain3/1
  Switch1/1 -> Integrator2/1

== system MPC_control_ID/Controllers/ECU ==
  <Accel> : Inport
  Acc to Torque Request : Gain  Gain=150
  MATLAB Function : MATLAB Function  TreatAsAtomicUnit=on
  Stop Simulation : Stop
  Trq Cmd : Outport
  wires:
  Acc to Torque Request/1 -> Trq Cmd/1
  <Accel>/1 -> MATLAB Function/1("input ")
  MATLAB Function/2(output) -> Stop Simulation/1
  MATLAB Function/1(input) -> Acc to Torque Request/1

== system MPC_control_ID/Controllers/Transmission Controller ==
  Acc : Inport
  EngSpd : Inport  Port=2  Unit=rad/s
  PropShaftSpd : Inport  Port=3
  10ms Function-Call Generator : simulink/Ports & Subsystems/Function-Call Generator  sample_time=Fcncal_transctrl_Ts  numberOfIterations=1
  Rate Transition{,1..3} (4 alike) : RateTransition
  Signal Specification : SignalSpecification  Unit=rpm
  TCM : Subsystem
  Unit Conversion : UnitConversion
  Gear : Outport
  wires:
  TCM/1(Gear Select) -> Rate Transition3/1
  Rate Transition/1 -> TCM/1(AccCmd)
  10ms Function-Call Generator/1 -> TCM/Trigger
  Acc/1 -> Rate Transition/1
  PropShaftSpd/1 -> Rate Transition2/1
  Rate Transition1/1 -> TCM/2(EngSpd)
  Rate Transition2/1 -> TCM/3(VehSpdFdbk)
  Rate Transition3/1 -> Gear/1
  Unit Conversion/1 -> Signal Specification/1
  Signal Specification/1 -> Rate Transition1/1  "EngSpd"
  EngSpd/1 -> Unit Conversion/1

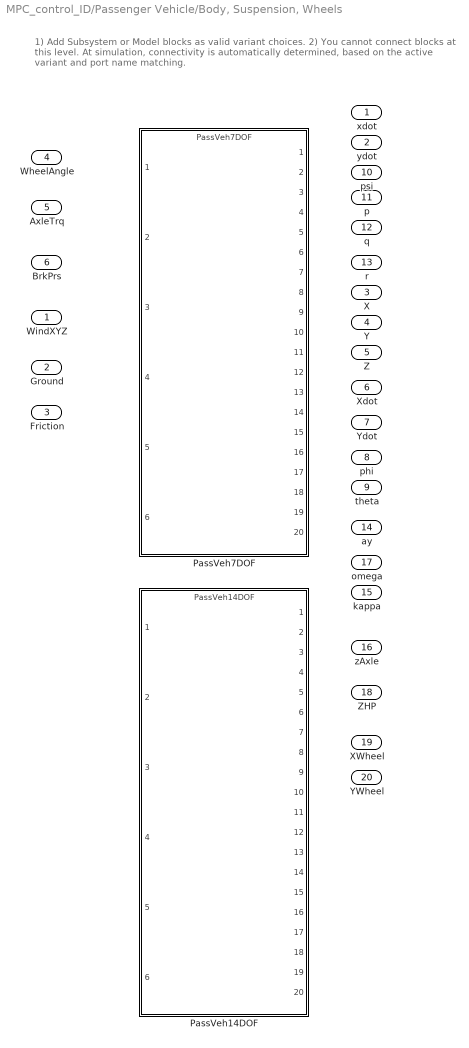
== system MPC_control_ID/Passenger Vehicle/Body, Suspension, Wheels ==
  note: 1) Add Subsystem or Model blocks as valid variant choices.
      | 2) You cannot connect blocks at this level. At simulation, connectivity is automatically
      | determined, based on the active variant and port name matching.
  WindXYZ : Inport
  Ground : Inport  Port=2  PortDimensions=4
  Friction : Inport  Port=3  PortDimensions=4
  WheelAngle : Inport  Port=4
  AxleTrq : Inport  Port=5
  BrkPrs : Inport  Port=6
  PassVeh14DOF : ModelReference  DisableCoverage=on  ModelNameDialog=PassVeh14DOF  VariantControl=3  ModelReferenceVersion=1.200
  PassVeh7DOF : ModelReference  DisableCoverage=on  ModelNameDialog=PassVeh7DOF  VariantControl=1  ModelReferenceVersion=1.152
  xdot : Outport
  ydot : Outport  Port=2
  X : Outport  Port=3
  Y : Outport  Port=4
  Z : Outport  Port=5
  Xdot : Outport  Port=6
  Ydot : Outport  Port=7
  phi : Outport  Port=8
  theta : Outport  Port=9
  psi : Outport  Port=10
  p : Outport  Port=11
  q : Outport  Port=12
  r : Outport  Port=13
  ay : Outport  Port=14
  kappa : Outport  Port=15
  zAxle : Outport  Port=16
  omega : Outport  Port=17
  ZHP : Outport  Port=18  Unit=m
  XWheel : Outport  Port=19
  YWheel : Outport  Port=20

== system MPC_control_ID/Passenger Vehicle/Engine ==
  note: 1) Add Subsystem or Model blocks as valid variant choices.
      | 2) You cannot connect blocks at this level. At simulation, connectivity is automatically
      | determined, based on the active variant and port name matching.
  TrqCmd : Inport
  EngSpd : Inport  Port=2  Unit=rad/s
  Ideal Mapped Engine : ModelReference  DisableCoverage=on  ModelNameDialog=SiMappedEngineV  VariantControl=0  ModelReferenceVersion=1.335
  EngTrq : Outport

== system MPC_control_ID/Passenger Vehicle/Steering, Transmission, Driveline and Brakes ==
  note: 1) Add Subsystem or Model blocks as valid variant choices.
      | 2) You cannot connect blocks at this level. At simulation, connectivity is automatically
      | determined, based on the active variant and port name matching.
  SteerHWCmd : Inport
  EngTrq : Inport  Port=2
  GearCmd : Inport  Port=3  OutDataTypeStr=int8
  BrkPrsCmd : Inport  Port=4  PortDimensions=4
  omega : Inport  Port=5
  Driveline Ideal Fixed Gear : ModelReference  DisableCoverage=on  ModelNameDialog=Driveline  VariantControl=0  ModelReferenceVersion=1.207
  WhlAng : Outport
  AxlTrq : Outport  Port=2
  BrkPrs : Outport  Port=3  PortDimensions=4
  EngSpd : Outport  Port=4  Unit=rad/s
  PropShftSpd : Outport  Port=5

== system MPC_control_ID/Passenger Vehicle/Subsystem ==
  Env : Inport
  Driveline : Inport  Port=2
  Bus Selector1 : BusSelector  OutputSignals=Gnd.z.G_FL_z,Gnd.z.G_FR_z,Gnd.z.G_RL_z,Gnd.z.G_RR_z
  Bus Selector2 : BusSelector  OutputSignals=Wind
  Bus Selector3 : BusSelector  OutputSignals=Gnd.mu.mu_FL,Gnd.mu.mu_FR,Gnd.mu.mu_RL,Gnd.mu.mu_RR
  Bus Selector4 : BusSelector  OutputSignals=WhlAng,AxlTrq,BrkPrs
  Vector Concatenate : Concatenate  NumInputs=4
  Vector Concatenate1 : Concatenate  NumInputs=4
  Wind : Outport
  Gnd : Outport  Port=2
  mu : Outport  Port=3
  WhlAng : Outport  Port=4
  AxleTrq : Outport  Port=5
  BrkPrs : Outport  Port=6
  wires:
  Env/1 -> Bus Selector3/1, Bus Selector1/1, Bus Selector2/1
  Bus Selector2/1 -> Wind/1  "<Wind>"
  Bus Selector3/1 -> Vector Concatenate/1  "<mu_FL>"
  Bus Selector3/2 -> Vector Concatenate/2  "<mu_FR>"
  Bus Selector3/3 -> Vector Concatenate/3  "<mu_RL>"
  Bus Selector3/4 -> Vector Concatenate/4  "<mu_RR>"
  Vector Concatenate/1 -> mu/1
  Bus Selector1/1 -> Vector Concatenate1/1  "<G_FL_z>"
  Bus Selector1/2 -> Vector Concatenate1/2  "<G_FR_z>"
  Bus Selector1/3 -> Vector Concatenate1/3  "<G_RL_z>"
  Bus Selector1/4 -> Vector Concatenate1/4  "<G_RR_z>"
  Vector Concatenate1/1 -> Gnd/1
  Driveline/1 -> Bus Selector4/1
  Bus Selector4/2 -> AxleTrq/1  "<AxlTrq>"
  Bus Selector4/1 -> WhlAng/1  "<WhlAng>"
  Bus Selector4/3 -> BrkPrs/1  "<BrkPrs>"

== system MPC_control_ID/Passenger Vehicle/Subsystem1 ==
  WhlAng : Inport
  AxlTrq : Inport  Port=2
  BrkPrs : Inport  Port=3
  EngSpd : Inport  Port=4
  PropShftSpd : Inport  Port=5
  Bus Creator1 : BusCreator  Inputs=5
  Driveline : Outport
  wires:
  Bus Creator1/1 -> Driveline/1  "Driveline"
  PropShftSpd/1 -> Bus Creator1/5  "PropShftSpd"
  AxlTrq/1 -> Bus Creator1/2  "AxlTrq"
  WhlAng/1 -> Bus Creator1/1  "WhlAng"
  EngSpd/1 -> Bus Creator1/4  "EngSpd"
  BrkPrs/1 -> Bus Creator1/3  "BrkPrs"

== system MPC_control_ID/Passenger Vehicle/Subsystem2 ==
  Cntrl : Inport
  SteerCmd : Inport  Port=2
  EngTrqCmd : Inport  Port=3
  Wheels : Inport  Port=4
  Bus Selector1 : BusSelector  OutputSignals=Steer
  Bus Selector2 : BusSelector  OutputSignals=omega
  Bus Selector3 : BusSelector  OutputSignals=Transmission.GearCmd,Brake.PrsCmd
  Bus Selector4 : BusSelector  OutputSignals=EngTrq
  Steer : Outport
  EngTrq : Outport  Port=2
  GearCmd : Outport  Port=3
  PrsCmd : Outport  Port=4
  omega : Outport  Port=5
  wires:
  Cntrl/1 -> Bus Selector3/1
  Bus Selector3/1 -> GearCmd/1  "<GearCmd>"
  SteerCmd/1 -> Bus Selector1/1
  Wheels/1 -> Bus Selector2/1
  Bus Selector2/1 -> omega/1  "<omega>"
  Bus Selector3/2 -> PrsCmd/1  "<PrsCmd>"
  EngTrqCmd/1 -> Bus Selector4/1
  Bus Selector1/1 -> Steer/1  "<Steer>"
  Bus Selector4/1 -> EngTrq/1  "<EngTrq>"

== system MPC_control_ID/Passenger Vehicle/Subsystem3 ==
  Cntrl : Inport
  Driveline : Inport  Port=2
  Bus Selector : BusSelector  OutputSignals=ECU.EngTrqCmd
  Bus Selector1 : BusSelector  OutputSignals=EngSpd
  EngTrqCmd : Outport
  EngSpd : Outport  Port=2
  wires:
  Driveline/1 -> Bus Selector1/1
  Cntrl/1 -> Bus Selector/1
  Bus Selector/1 -> EngTrqCmd/1  "<EngTrqCmd>"
  Bus Selector1/1 -> EngSpd/1  "<EngSpd>"

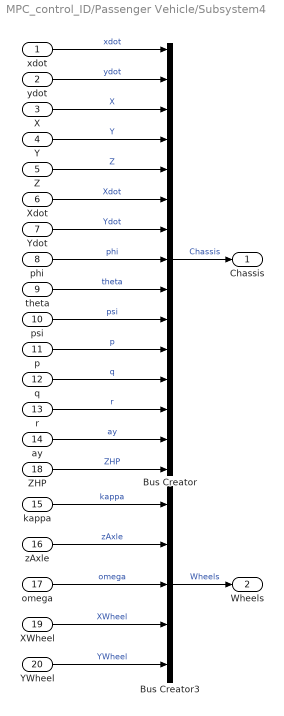
== system MPC_control_ID/Passenger Vehicle/Subsystem4 ==
  xdot : Inport
  ydot : Inport  Port=2
  X : Inport  Port=3
  Y : Inport  Port=4
  Z : Inport  Port=5
  Xdot : Inport  Port=6
  Ydot : Inport  Port=7
  phi : Inport  Port=8
  theta : Inport  Port=9
  psi : Inport  Port=10
  p : Inport  Port=11
  q : Inport  Port=12
  r : Inport  Port=13
  ay : Inport  Port=14
  kappa : Inport  Port=15
  zAxle : Inport  Port=16
  omega : Inport  Port=17
  ZHP : Inport  Port=18
  XWheel : Inport  Port=19
  YWheel : Inport  Port=20
  Bus Creator : BusCreator  Inputs=15
  Bus Creator3 : BusCreator  Inputs=5
  Chassis : Outport
  Wheels : Outport  Port=2
  wires:
  X/1 -> Bus Creator/3  "X"
  psi/1 -> Bus Creator/10  "psi"
  ydot/1 -> Bus Creator/2  "ydot"
  Z/1 -> Bus Creator/5  "Z"
  Bus Creator/1 -> Chassis/1  "Chassis"
  Y/1 -> Bus Creator/4  "Y"
  xdot/1 -> Bus Creator/1  "xdot"
  r/1 -> Bus Creator/13  "r"
  ay/1 -> Bus Creator/14  "ay"
  omega/1 -> Bus Creator3/3  "omega"
  zAxle/1 -> Bus Creator3/2  "zAxle"
  kappa/1 -> Bus Creator3/1  "kappa"
  Bus Creator3/1 -> Wheels/1  "Wheels"
  theta/1 -> Bus Creator/9  "theta"
  phi/1 -> Bus Creator/8  "phi"
  Xdot/1 -> Bus Creator/6  "Xdot"
  Ydot/1 -> Bus Creator/7  "Ydot"
  ZHP/1 -> Bus Creator/15  "ZHP"
  p/1 -> Bus Creator/11  "p"
  q/1 -> Bus Creator/12  "q"
  YWheel/1 -> Bus Creator3/5  "YWheel"
  XWheel/1 -> Bus Creator3/4  "XWheel"

== system MPC_control_ID/Passenger Vehicle/Subsystem5 ==
  "EngTrq " : Inport
  Bus Creator : BusCreator  Inputs=1
  Eng : Outport
  wires:
  "EngTrq "/1 -> Bus Creator/1  "EngTrq"
  Bus Creator/1 -> Eng/1

== system MPC_control_ID/Visualization/3D Engine ==
  note: 1) Add Subsystem or Model blocks as valid variant choices.
      | 2) You cannot connect blocks at this level. At simulation, connectivity is automatically
      | determined, based on the active variant and port name matching.
  VehFdbk : Inport
  3D Engine : Subsystem  VariantControl=1
  3D Engine Disabled : Subsystem  VariantControl=0

== system MPC_control_ID/Visualization/Acceleration Cmd ==

== system MPC_control_ID/Visualization/Brake Cmd ==

== system MPC_control_ID/Visualization/Engine Tach [rpm] ==

== system MPC_control_ID/Visualization/Handwheel Angle [deg] ==

== system MPC_control_ID/Visualization/Lateral Acceleration [g] ==

== system MPC_control_ID/Visualization/Speed [mph] ==

== system MPC_control_ID/Visualization/Vehicle XY Plotter ==
  VehFdbk : Inport
  Bus Selector1 : BusSelector  OutputSignals=Body.phi,Body.theta,Body.psi  OutputAsBus=on
  Bus Selector2 : BusSelector  OutputSignals=Driveline.WhlAng  OutputAsBus=on
  Bus Selector3 : BusSelector  OutputSignals=Body.X,Body.Y,Body.Z  OutputAsBus=on
  Bus Selector4 : BusSelector  OutputSignals=Body.Xdot,Body.Ydot  OutputAsBus=on
  Bus to Vector{,1..3} (4 alike) : BusToVector
  Ground : Ground
  Rate Transition{1..2,5..6} (4 alike) : RateTransition  OutPortSampleTime=pltDT
  Vector Concatenate : Concatenate
  Vehicle XY Plotter : vehdynlibviscommon/Vehicle XY Plotter  bufferSize=bufferSize  w=w  a=a  b=b
  wires:
  Bus to Vector2/1 -> Rate Transition1/1  "InertCGDisp"
  Rate Transition5/1 -> Vehicle XY Plotter/1
  Bus Selector4/1 -> Bus to Vector1/1
  Rate Transition1/1 -> Vehicle XY Plotter/2
  Rate Transition6/1 -> Vehicle XY Plotter/3
  Vector Concatenate/1 -> Rate Transition6/1  "InertCGVel"
  Bus Selector1/1 -> Bus to Vector2/1
  Bus to Vector/1 -> Rate Transition5/1  "InertCGDisp"
  Bus Selector3/1 -> Bus to Vector/1
  Bus to Vector1/1 -> Vector Concatenate/1
  Ground/1 -> Vector Concatenate/2
  Bus to Vector3/1 -> Rate Transition2/1
  Bus Selector2/1 -> Bus to Vector3/1
  VehFdbk/1 -> Bus Selector1/1, Bus Selector2/1, Bus Selector4/1, Bus Selector3/1
  Rate Transition2/1 -> Vehicle XY Plotter/4

== system MPC_control_ID/Controllers/Brake Controller/Brake Pressure Control ==
  note: 1) Add Subsystem or Model blocks as valid variant choices.
      | 2) You cannot connect blocks at this level. At simulation, connectivity is automatically
      | determined, based on the active variant and port name matching.
  Pref : Inport
  xdot : Inport  Port=2
  <Kappa> : Inport  Port=3
  Bang Bang ABS : Subsystem  VariantControl=1
  Open Loop : Subsystem  VariantControl=0
  PCmd : Outport

== system MPC_control_ID/Controllers/Transmission Controller/TCM ==
  AccCmd : Inport
  EngSpd : Inport  Port=2
  VehSpdFdbk : Inport  Port=3
  function : TriggerPort  TriggerType=function-call  VariantControl=Variant
  Neutral Select : Subsystem
  Prop Shaft Speed LPF : DiscreteTransferFcn  Numerator=[0.000000000000000 0.009950166250832 ]  Denominator=[1.000000000000000 -0.990049833749168 ]  mask(DiscretizedDiscreteTransferFcn){}
      mask init:
      | %zoh
  TCM Shift Controller : Stateflow chart  TreatAsAtomicUnit=on
  prop speed to vehicle speed : Gain  Gain=0.45
  Gear Select : Outport
  wires:
  VehSpdFdbk/1 -> Prop Shaft Speed LPF/1
  TCM Shift Controller/1(GearState) -> Gear Select/1  "GearCmd"
  AccCmd/1 -> Neutral Select/1(AccCmd), TCM Shift Controller/2(pedal)  "AccCmd"
  Neutral Select/1(Neutral Select) -> TCM Shift Controller/3(Neutral)
  EngSpd/1 -> Neutral Select/2(EngSpd)
  prop speed to vehicle speed/1 -> TCM Shift Controller/1(speed)
  Prop Shaft Speed LPF/1 -> prop speed to vehicle speed/1

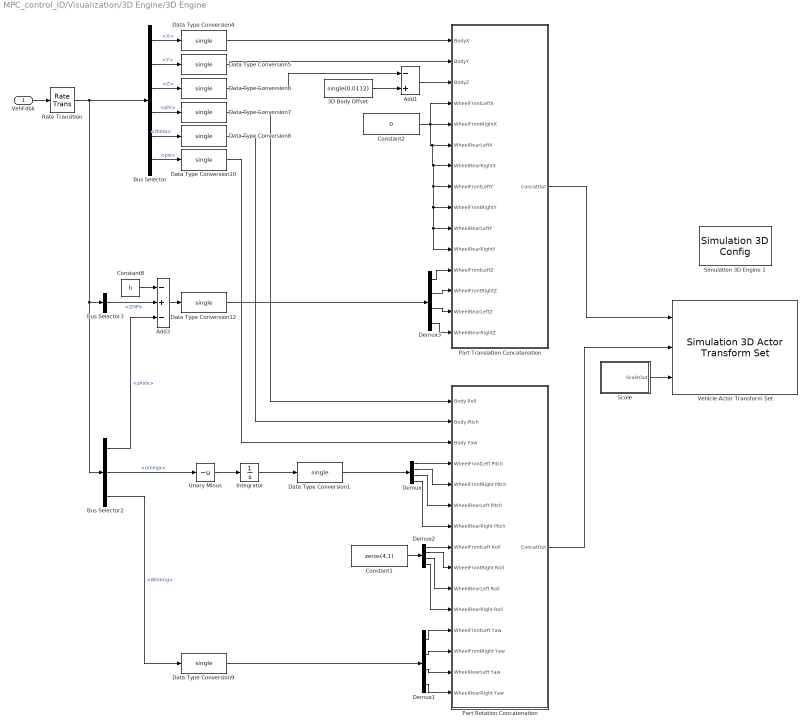
== system MPC_control_ID/Visualization/3D Engine/3D Engine ==
  VehFdbk : Inport
  3D Body Offset : Constant  Value=single(0.0112)  OutDataTypeStr=single
  Add1 : Sum  Inputs=-+
  Add3 : Sum  Inputs=-+-
  Bus Selector : BusSelector  OutputSignals=Body.X,Body.Y,Body.Z,Body.phi,Body.theta,Body.psi
  Bus Selector2 : BusSelector  OutputSignals=Wheels.zAxle,Wheels.omega,Driveline.WhlAng
  Bus Selector3 : BusSelector  OutputSignals=Body.ZHP
  Constant1 : Constant  Value=zeros(4,1)  OutDataTypeStr=single
  Constant2 : Constant  Value=0  OutDataTypeStr=single
  Constant8 : Constant  Value=h
  Data Type Conversion{1,4..10,12} (9 alike) : DataTypeConversion  OutDataTypeStr=single
  Demux{,1..3} (4 alike) : Demux
  Integrator : Integrator  WrapState=on  WrappedStateUpperValue=2*pi  WrappedStateLowerValue=0  ZeroCross=off
  Part Rotation Concatenation : Subsystem
  Part Translation Concatenation : Subsystem
  Rate Transition : RateTransition  OutPortSampleTime=dt3D
  Scale : Subsystem
  Simulation 3D Engine 1 : sim3dlib/Simulation 3D Config  Priority=1  ProjectFormat=Executable  ProjectName=VehicleSimulation.exe  SceneDesc=Straight road  OpVisEn=off  Ts=dt3D
      settings: AttributesFormatString=Priority: %<Priority>
  Unary Minus : UnaryMinus
  Vehicle Actor Transform Set : sim3dlib/Simulation 3D Actor Transform Set  ActorTag=SimulinkVehicle1  ActorType=Passenger vehicle  PassVehMesh=Muscle car  VehColor=Red  NumberOfParts=5  CustNumOfParts=3  Translation=[0 0 1; 0 0 0; 0 0 0; 0 0 0; 0 0 0]  Rotation=[0 0 0; 0 0 0; 0 0 0; 0 0 0; 0 0 0]  Scale=[1 1 1; 1 1 1; 1 1 1; 1 1 1; 1 1 1]  Ts=dt3D
  wires:
  Unary Minus/1 -> Integrator/1
  Bus Selector3/1 -> Add3/2  "<ZHP>"
  Add3/1 -> Data Type Conversion12/1
  Bus Selector2/1 -> Add3/3  "<zAxle>"
  Constant8/1 -> Add3/1
  Rate Transition/1 -> Bus Selector/1, Bus Selector3/1, Bus Selector2/1
  Scale/1(ScaleOut) -> Vehicle Actor Transform Set/3
  Demux/4 -> Part Rotation Concatenation/7(WheelRearRight Ptich)
  Demux/3 -> Part Rotation Concatenation/6(WheelRearLeft Pitch)
  Demux/2 -> Part Rotation Concatenation/5(WheelFrontRight Pitch)
  Demux/1 -> Part Rotation Concatenation/4(WheelFrontLeft Pitch)
  Constant1/1 -> Demux2/1
  Bus Selector/4 -> Data Type Conversion7/1  "<phi>"
  Data Type Conversion6/1 -> Add1/1
  Part Rotation Concatenation/1(ConcatOut) -> Vehicle Actor Transform Set/2
  Part Translation Concatenation/1(ConcatOut) -> Vehicle Actor Transform Set/1
  Data Type Conversion12/1 -> Demux3/1
  Demux3/4 -> Part Translation Concatenation/15(WheelRearRightZ)
  Demux3/3 -> Part Translation Concatenation/14(WheelRearLeftZ)
  Demux3/1 -> Part Translation Concatenation/12(WheelFrontLeftZ)
  Demux3/2 -> Part Translation Concatenation/13(WheelFrontRightZ)
  VehFdbk/1 -> Rate Transition/1
  Add1/1 -> Part Translation Concatenation/3(BodyZ)
  3D Body Offset/1 -> Add1/2
  Demux1/4 -> Part Rotation Concatenation/15(WheelRearRight Yaw)
  Demux1/3 -> Part Rotation Concatenation/14(WheelRearLeft Yaw)
  Demux2/1 -> Part Rotation Concatenation/8(WheelFrontLeft Roll)
  Demux2/2 -> Part Rotation Concatenation/9(WheelFrontRight Roll)
  Demux2/3 -> Part Rotation Concatenation/10(WheelRearLeft Roll)
  Demux2/4 -> Part Rotation Concatenation/11(WheelRearRight Roll)
  Bus Selector2/3 -> Data Type Conversion9/1  "<WhlAng>"
  Bus Selector2/2 -> Unary Minus/1  "<omega>"
  Data Type Conversion9/1 -> Demux1/1
  Demux1/1 -> Part Rotation Concatenation/12(WheelFrontLeft Yaw)
  Demux1/2 -> Part Rotation Concatenation/13(WheelFrontRight Yaw)
  Integrator/1 -> Data Type Conversion1/1
  Data Type Conversion1/1 -> Demux/1
  Data Type Conversion8/1 -> Part Rotation Concatenation/2(Body Ptich)
  Data Type Conversion5/1 -> Part Translation Concatenation/2(BodyY)
  Data Type Conversion10/1 -> Part Rotation Concatenation/3(Body Yaw)
  Constant2/1 -> Part Translation Concatenation/5(WheelFrontRightX), Part Translation Concatenation/6(WheelRearLeftX), Part Translation Concatenation/7(WheelRearRightX), Part Translation Concatenation/8(WheelFrontLeftY), Part Translation Concatenation/9(WheelFrontRightY), Part Translation Concatenation/10(WheelRearLeftY), Part Translation Concatenation/11(WheelRearRightY), Part Translation Concatenation/4(WheelFrontLeftX)
  Data Type Conversion4/1 -> Part Translation Concatenation/1(BodyX)
  Data Type Conversion7/1 -> Part Rotation Concatenation/1(Body Roll)
  Bus Selector/1 -> Data Type Conversion4/1  "<X>"
  Bus Selector/2 -> Data Type Conversion5/1  "<Y>"
  Bus Selector/3 -> Data Type Conversion6/1  "<Z>"
  Bus Selector/6 -> Data Type Conversion10/1  "<psi>"
  Bus Selector/5 -> Data Type Conversion8/1  "<theta>"

== system MPC_control_ID/Visualization/3D Engine/3D Engine Disabled ==
  VehFdbk : Inport
  Terminator : Terminator
  wires:
  VehFdbk/1 -> Terminator/1

== system MPC_control_ID/Controllers/Brake Controller/Brake Pressure Control/Bang Bang ABS ==
  Pref : Inport
  xdot : Inport  Port=2
  <Kappa> : Inport  Port=3
  Abs : Abs
  Add : Sum  Inputs=-+
  Bang-bang controller : Subsystem  mask(Sign){}
      mask help: y = sign(x)
      mask Help: Sign Function:\n\t\t\ty = 1 if x > 0\n\t\t\ty = 0 if x = 0\n\t\t\ty = -1 if x < 0
      mask Display: plot(-50,-50,50,50,[-50,50],[0,0],[0,0],[-50,50],[-40,0],[-30,-30],[0,40],[30,30])
  Compare To Constant : simulink/Logic and Bit Operations/Compare To Constant  relop=>=  const=.2  OutDataTypeStr=boolean
  Compare To Constant1 : simulink/Logic and Bit Operations/Compare To Constant  relop=>=  const=.75  OutDataTypeStr=boolean
  Compare To Constant2 : simulink/Logic and Bit Operations/Compare To Constant  relop=>=  const=.5  OutDataTypeStr=boolean
  Constant : Constant  Value=.25
  Debounce : autolibutils/Debounce  DbcOn_Cnts=.1*.001  DbcOff_Cnts=.1*.001  aMode=aMode
      settings: SourceProductName=Powertrain Blockset  SourceProductBaseCode=PW
  Gain : Gain  Gain=200
  Logical Operator : Logic  Inputs=3  AllPortsSameDT=off  OutDataTypeStr=boolean
  Rate Transition : RateTransition  OutPortSampleTime=.001
  Rate Transition1 : RateTransition
  Switch : Switch  Criteria=u2 > Threshold  ZeroCross=off
  PCmd : Outport
  wires:
  Bang-bang controller/1(out_1) -> Gain/1
  Add/1 -> Bang-bang controller/1(in_1)
  Rate Transition1/1 -> PCmd/1
  <Kappa>/1 -> Rate Transition/1
  Pref/1 -> Switch/3, Compare To Constant1/1  "Pref"
  Constant/1 -> Add/2  "slip ref"
  Switch/1 -> Rate Transition1/1
  Rate Transition/1 -> Add/1, Compare To Constant/1
  Logical Operator/1 -> Debounce/1
  Compare To Constant/1 -> Logical Operator/2
  Compare To Constant1/1 -> Logical Operator/3
  Debounce/1 -> Switch/2
  xdot/1 -> Abs/1
  Abs/1 -> Compare To Constant2/1
  Compare To Constant2/1 -> Logical Operator/1
  Gain/1 -> Switch/1

== system MPC_control_ID/Controllers/Brake Controller/Brake Pressure Control/Open Loop ==
  Pref : Inport
  PCmd : Outport
  wires:
  Pref/1 -> PCmd/1  "Reference Slip"

== system MPC_control_ID/Controllers/Transmission Controller/TCM/Neutral Select ==
  AccCmd : Inport
  EngSpd : Inport  Port=2
  Constant : Constant  Value=1200
  Constant1 : Constant  Value=1e-6
  Logical Operator : Logic  AllPortsSameDT=off  OutDataTypeStr=boolean
  Relational Operator : RelationalOperator  Operator=<=  OutDataTypeStr=boolean  RndMeth=Simplest
  Relational Operator1 : RelationalOperator  Operator=<=  OutDataTypeStr=boolean  RndMeth=Simplest
  Saturation1 : Saturate  UpperLimit=10e3  LowerLimit=0
  rad/s to RPM : Gain  Gain=30/pi
  Neutral Select : Outport
  wires:
  Saturation1/1 -> Relational Operator/1
  Relational Operator1/1 -> Logical Operator/1
  AccCmd/1 -> Relational Operator1/1
  Constant1/1 -> Relational Operator1/2
  Logical Operator/1 -> Neutral Select/1
  Constant/1 -> Relational Operator/2
  Relational Operator/1 -> Logical Operator/2
  rad/s to RPM/1 -> Saturation1/1
  EngSpd/1 -> rad/s to RPM/1
